simulink model "proceso"  (R2018a)
settings: Solver=VariableStepAuto  StartTime=0.0  StopTime=3000  RelTol=1e-3
values from neighbouring files (symbols this model uses):
  Ad = [0.9888    0.0001    0.0112 ... (first row only)    [proceso.m]
  Bd = [64.5687    0.0014 ... (first row only)    [proceso.m]
  Cd = eye(3)    [codigo_ex.m]    (also in sistema_tanques_control.m; tank_mod.m)
  h_max = 0.62    [codigo_ex.m]    (also in sistema_tanques_control.m; tank_mod.m)
  h_min = 0    [codigo_ex.m]    (also in sistema_tanques_control.m; tank_mod.m)
  tm = 1    [codigo_ex.m]    (also in sistema_tanques_control.m; tank_mod.m)
settings Model: Creator=carma  LastModifiedBy=carma

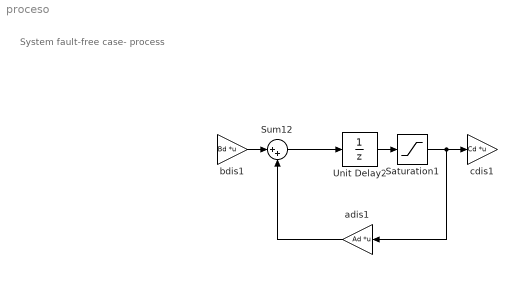
== system proceso ==
  note: System fault-free case- process
  Saturation1 : Saturate  UpperLimit=h_max  LowerLimit=h_min
  Sum12 : Sum  Inputs=|++  SampleTime=tm
  Unit Delay2 : UnitDelay  SampleTime=tm
  adis1 : Gain  Gain=Ad  Multiplication=Matrix(K*u) (u vector)  SampleTime=tm
  bdis1 : Gain  Gain=Bd  Multiplication=Matrix(K*u) (u vector)  SampleTime=tm
  cdis1 : Gain  Gain=Cd  Multiplication=Matrix(K*u) (u vector)  SampleTime=tm
  wires:
  Sum12/1 -> Unit Delay2/1
  ? -> bdis1/1
  Unit Delay2/1 -> Saturation1/1
  adis1/1 -> Sum12/2
  bdis1/1 -> Sum12/1
  Saturation1/1 -> adis1/1, cdis1/1
